simulink model "HEV"  (R2023b)
settings: Solver=ode1  StartTime=0.0  StopTime=1800  FixedStep=1  RelTol=1e-3
undefined symbols (not defined in the file): alpha_em, eta_EM_mapG, eta_EM_mapM, gamma, gamma_fd, Paux_em, T_EM_max, theta_EM, Tsplit_em, w_EM_row, w_EM_upper, w_shift
libraries: EnergyStorage x2, EnergyConverters x1, DrivingCycle x1, GearSystems x1, GearSystemsControl x1, VehicleBody x1
settings Model: Creator=dadikozyanaa  LastModifiedBy=koenjacobs
settings DebuggingCC: UnconnectedInputMsg=warning  UnconnectedOutputMsg=warning  UnconnectedLineMsg=warning
settings ModelReferenceCC: EnableRefExpFcnMdlSchedulingChecks=on
settings RTWCC: DLArmComputeVersion=19.05

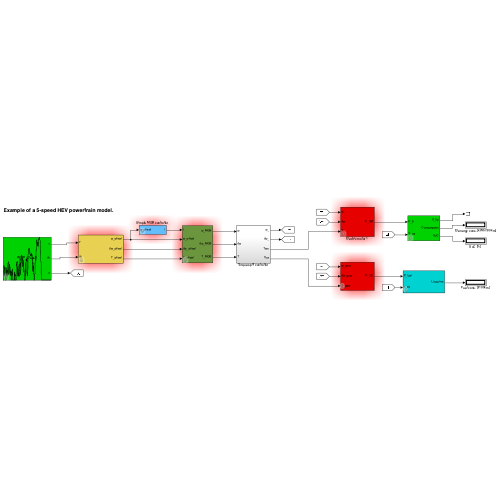
[thumbnail: Simulink's stored preview of the top-level diagram]
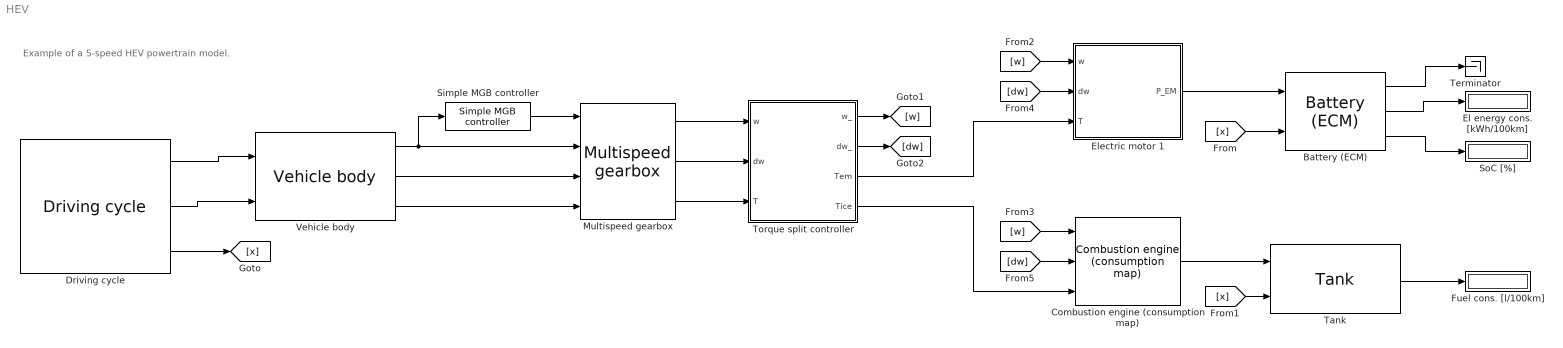
== system HEV ==
  note: Example of a 5-speed HEV powertrain model.
  Battery (ECM) : EnergyStorage/Battery (ECM)  BattType=High Energy  BattChem=NMC  init_SoC=50  bt_Np=Np  bt_Ns=100  SoC_low=10  SoC_high=90  U_cell=3.7  Capacity=2.6  CellWeight=46.5  bt_vol=370  bt_cap=91  bt_weight=162.75
      settings: SourceProductName=QSS TU/e Toolbox
  Combustion engine (consumption map) : EnergyConverters/Combustion engine  (consumption map)  Tag=combustion engine  enginetype=Spark ignition  enginenumberCI=37kW  enginenumberSI=102kW  P_aux=Paux_ice  ENABLE_FUEL_CUTOFF=on  T_CE_cutoff=Tcutoff_ice  P_CE_cutoff=Pcutoff_ice  scale_CE=alpha_ice
      settings: SourceProductName=QSS TU/e Toolbox
  Driving cycle : DrivingCycle/Driving cycle  bool_combine=off  cyclenr=Europe: WLTP Class 3  cyclenr2=Europe: EUDC  gradient_speed=80  cyclerep=1  stepsize=1  autostop=on  slope_bool_cycle=on  mode_bool=off  mode_array=0
      settings: SourceProductName=QSS TU/e Toolbox
  El energy cons. [kWh/100km] : Display
  Electric motor 1 : Subsystem  mask(Electric Motor){motortype=Permanet magnet, motornumberPM=33 kW, motornumberAC=25 kW, scale_EM=alpha_em, P_aux=Paux_em, motornumberSim=1}
      mask prompts: motortype "Select electric machine type:"; motornumberPM "Select electric machine model:"; motornumberAC "Select electric machine model:"; scale_EM "Motor scaling factor [-]:"; P_aux "Auxiliary power [W]:"; motornumberSim "Select electric machine number:"
      mask help:
      | This block simulates the behaviour of an electric motor. The block is based on an efficiency map.
      |
      | Input:
      | =====
      | 	w_gear	Speed of the fly wheel [rad/s]
      | 	dw_gear	Acceleration of the fly wheel [rad/s^2]
      | 	T_gear	Torque on the fly wheel [Nm]
      |
      | Output:
      | ======
      | 	P_EM	Power produced by the EM [W]
      mask init:
      | init_EM;
      mask Help: web(which('help_ElectricMotor.html'), '-helpbrowser')
      mask TypeOptions motortype: Permanet magnet | Induction (AC)
      mask Callback motortype:
      | maskStr = get_param(gcb,'motortype');
      | 
      | switch maskStr
      |     case 'Permanet magnet'
      |         set_param(gcb,'MaskVisibilities',{'on';'on';'off';'on';'on';'on'}),
      |     case 'Induction (AC)'
      |         set_param(gcb,'MaskVisibilities',{'on';'off';'on';'on';'on';'on'}),
      | end
      mask TypeOptions motornumberPM: 8 kW | 15 kW LYNX | 16 kW | 16 kW EVS | 23 kW | 25 kW | 30 kW Prius | 32 kW | 32 kW EV | 32 kW EVS | 33 kW | 49 kW | 58 kW | 63 kW | 100 kW
      mask TypeOptions motornumberAC: 25 kW | 30 kW | 59 kW | 62 kW | 75 kW | 83 kW | 124 kW | 150 kW | 187 kW
      mask TypeOptions motornumberSim: 1 | 2 | 3 | 4 | 5 | 6 | 7 | 8
      mask DialogControl ParameterGroupVar Prompt: EM type and model
      mask DialogControl Container3 Prompt: Parameters
      mask DialogControl ParameterGroupVar_copy Prompt: EM number
      mask Display:
      | %disp(messageEM, 'texmode', 'on')
      | %plot(w_EM_max, T_EM_max);
  Fuel cons. [l/100km] : Display
  Multispeed gearbox : GearSystems/Multispeed gearbox  Tag=transmission  nr_gears=5  i_1=gamma(1)  i_2=gamma(2)  i_3=gamma(3)  i_4=gamma(4)  i_5=gamma(5)  i_6=2.748  i_diff=gamma_fd  e_GT=e_gb  P_GT0=Ploss  w_wheel_min=wem_min
      settings: SourceProductName=QSS TU/e Toolbox
  Simple MGB controller : GearSystemsControl/Simple MGB controller  nr_gears=5  w_shift2=w_shift/gamma(1)/gamma_fd  w_shift3=w_shift/gamma(2)/gamma_fd  w_shift4=w_shift/gamma(3)/gamma_fd  w_shift5=w_shift/gamma(4)/gamma_fd  w_shift6=1e10
      settings: SourceProductName=QSS TU/e Toolbox
  SoC [%] : Display
  Tank : EnergyStorage/Tank  Tag=tank  fuel=Gasoline  flag_cold_start=on
      settings: SourceProductName=QSS TU/e Toolbox
  Terminator : Terminator
  Torque split controller : Subsystem
  Vehicle body : VehicleBody/Vehicle body  drivetype=FWD  m_f=mv  mt2m_f=J_rot  A_f=Af  d_wheel=dw  cw=cd  mu=cr
      settings: SourceProductName=QSS TU/e Toolbox
  wires:
  Driving cycle/1 -> Vehicle body/1
  Driving cycle/2 -> Vehicle body/2
  Tank/1 -> Fuel cons. [l/100km]/1
  Combustion engine (consumption map)/1 -> Tank/1
  Vehicle body/1 -> Simple MGB controller/1, Multispeed gearbox/2
  Simple MGB controller/1 -> Multispeed gearbox/1
  Vehicle body/2 -> Multispeed gearbox/3
  Vehicle body/3 -> Multispeed gearbox/4
  Battery (ECM)/2 -> El energy cons. [kWh/100km]/1
  Electric motor 1/1(P_EM) -> Battery (ECM)/1
  Battery (ECM)/3 -> SoC [%]/1
  Multispeed gearbox/2 -> Torque split controller/2(dw)
  Multispeed gearbox/3 -> Torque split controller/3(T)
  [x] -> Battery (ECM)/2
  [x] -> Tank/2
  Torque split controller/1(w_) -> [w]
  Torque split controller/2(dw_) -> [dw]
  [w] -> Electric motor 1/1(w)
  [w] -> Combustion engine (consumption map)/1
  [dw] -> Electric motor 1/2(dw)
  [dw] -> Combustion engine (consumption map)/2
  Torque split controller/3(Tem) -> Electric motor 1/3(T)
  Torque split controller/4(Tice) -> Combustion engine (consumption map)/3
  Multispeed gearbox/1 -> Torque split controller/1(w)
  Driving cycle/3 -> [x]
  Battery (ECM)/1 -> Terminator/1

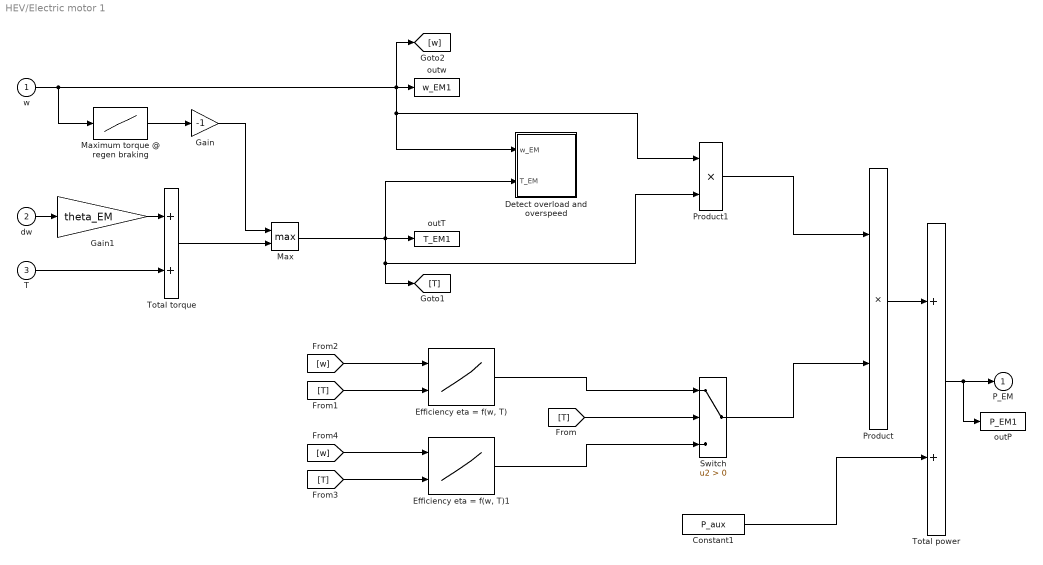
== system HEV/Electric motor 1 ==
  w : Inport
  dw : Inport  Port=2
  T : Inport  Port=3
  Constant1 : Constant  Value=P_aux
  Detect overload and overspeed : Subsystem
  "Efficiency eta = f(w, T)" : Lookup2D  RowIndex=w_EM_row  ColumnIndex=T_EM_col  Table=eta_EM_mapM  SaturateOnIntegerOverflow=off  InputSameDT=off
  "Efficiency eta = f(w, T)1" : Lookup2D  RowIndex=w_EM_row  ColumnIndex=T_EM_col  Table=eta_EM_mapG  SaturateOnIntegerOverflow=off  InputSameDT=off
  Gain : Gain  Gain=-1
  Gain1 : Gain  Gain=theta_EM  SaturateOnIntegerOverflow=on  OutDataTypeStr=Inherit: Same as input  ParamDataTypeStr=Inherit: Same as input
  Max : MinMax  Function=max  Inputs=2
  Maximum torque @ regen braking : Lookup  InputValues=w_EM_row  Table=T_EM_max
  Product : Product  InputSameDT=on  RndMeth=Zero  SaturateOnIntegerOverflow=on  OutDataTypeStr=Inherit: Same as first input
  Product1 : Product
  Switch : Switch  Criteria=u2 > Threshold  SaturateOnIntegerOverflow=off  InputSameDT=off
  Total power : Sum  InputSameDT=on  SaturateOnIntegerOverflow=on  OutDataTypeStr=Inherit: Same as first input
  Total torque : Sum  InputSameDT=on  SaturateOnIntegerOverflow=on  OutDataTypeStr=Inherit: Same as first input
  outP : ToWorkspace  VariableName=P_EM1  SampleTime=-1
  outT : ToWorkspace  VariableName=T_EM1  SampleTime=-1
  outw : ToWorkspace  VariableName=w_EM1  SampleTime=-1
  P_EM : Outport  InitialOutput=0
  wires:
  Gain/1 -> Max/1
  Max/1 -> [T], Product1/2, outT/1, Detect overload and overspeed/2(T_EM)
  Total torque/1 -> Max/2
  Maximum torque @ regen braking/1 -> Gain/1
  Switch/1 -> Product/2
  Product1/1 -> Product/1
  [T] -> "Efficiency eta = f(w, T)1"/2
  [w] -> "Efficiency eta = f(w, T)1"/1
  [T] -> "Efficiency eta = f(w, T)"/2
  [w] -> "Efficiency eta = f(w, T)"/1
  "Efficiency eta = f(w, T)1"/1 -> Switch/3
  "Efficiency eta = f(w, T)"/1 -> Switch/1
  [T] -> Switch/2
  w/1 -> outw/1, [w], Detect overload and overspeed/1(w_EM), Product1/1, Maximum torque @ regen braking/1
  dw/1 -> Gain1/1
  T/1 -> Total torque/2
  Gain1/1 -> Total torque/1
  Constant1/1 -> Total power/2
  Product/1 -> Total power/1
  Total power/1 -> outP/1, P_EM/1

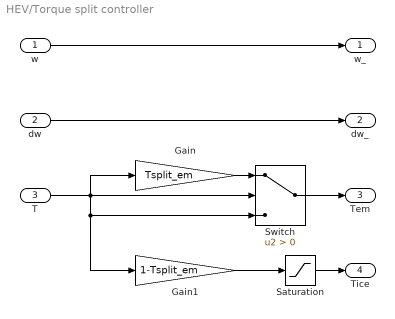
== system HEV/Torque split controller ==
  w : Inport
  dw : Inport  Port=2
  T : Inport  Port=3
  Gain : Gain  Gain=Tsplit_em
  Gain1 : Gain  Gain=1-Tsplit_em
  Saturation : Saturate  UpperLimit=inf  LowerLimit=0
  Switch : Switch  Criteria=u2 > Threshold  SaturateOnIntegerOverflow=off  InputSameDT=off
  w_ : Outport
  dw_ : Outport  Port=2
  Tem : Outport  Port=3
  Tice : Outport  Port=4
  wires:
  w/1 -> w_/1
  dw/1 -> dw_/1
  T/1 -> Gain/1, Switch/2, Switch/3, Gain1/1
  Gain/1 -> Switch/1
  Gain1/1 -> Saturation/1
  Saturation/1 -> Tice/1
  Switch/1 -> Tem/1

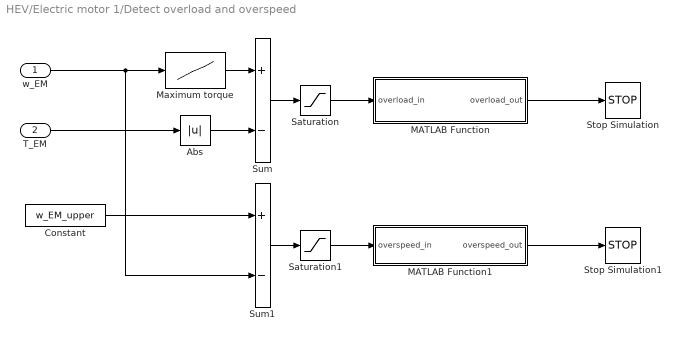
== system HEV/Electric motor 1/Detect overload and overspeed ==
  w_EM : Inport
  T_EM : Inport  Port=2
  Abs : Abs
  Constant : Constant  Value=w_EM_upper
  MATLAB Function : MATLAB Function  TreatAsAtomicUnit=on
  MATLAB Function1 : MATLAB Function  TreatAsAtomicUnit=on
  Maximum torque : Lookup  InputValues=w_EM_row  Table=T_EM_max
  Saturation : Saturate  UpperLimit=0  LowerLimit=-inf
  Saturation1 : Saturate  UpperLimit=0  LowerLimit=-inf
  Stop Simulation : Stop
  Stop Simulation1 : Stop
  Sum : Sum  Inputs=+-  InputSameDT=on  SaturateOnIntegerOverflow=on  OutDataTypeStr=Inherit: Same as first input
  Sum1 : Sum  Inputs=+-  InputSameDT=on  SaturateOnIntegerOverflow=on  OutDataTypeStr=Inherit: Same as first input
  wires:
  Saturation1/1 -> MATLAB Function1/1(overspeed_in)
  Sum1/1 -> Saturation1/1
  Constant/1 -> Sum1/1
  Saturation/1 -> MATLAB Function/1(overload_in)
  Abs/1 -> Sum/2
  Maximum torque/1 -> Sum/1
  T_EM/1 -> Abs/1
  w_EM/1 -> Sum1/2, Maximum torque/1
  Sum/1 -> Saturation/1
  MATLAB Function/1(overload_out) -> Stop Simulation/1
  MATLAB Function1/1(overspeed_out) -> Stop Simulation1/1

== matlab function HEV/Electric motor 1/Detect overload and overspeed/MATLAB Function1 ==
  data: overspeed_in input; overspeed_out output
function overspeed_out = overspeed_fnc(overspeed_in)

if overspeed_in~=0
     disp('Simulation stopped due to Motor Overspeed.')
end

overspeed_out = overspeed_in;

== matlab function HEV/Electric motor 1/Detect overload and overspeed/MATLAB Function ==
  data: overload_in input; overload_out output
function overload_out = overload_fnc(overload_in)

if overload_in~=0
    disp('Simulation stopped due to Motor Overload.')
end

overload_out = overload_in;
